simulink model "KPA_ALL"  (R2022b)
settings: Solver=FixedStepAuto  StartTime=0.0  StopTime=1  RelTol=1e-3
model workspace (MAT data in the model file):
  OutputBufferSize = 2
  OutputSampesPerSymbol = 4
  OutputSamplesPerSymbol = 4
  SNR = 16
  SampleTimeGenerator = 2.5e-06
undefined symbols (not defined in the file or in its folder): Add, DiscIntNeverNeededParam, magnitude, Shift
libraries: hdlsllib x16, simulink x5, commhdlcrc x3, commdigbbndpm3 x2, commfilt2 x2, commdigbbndam3 x2, commchan3 x1, commseqgen3 x1, commrandsrc3 x1, commsync2 x1, commsink2 x1, commutil2 x1
(part 1 of 2)
settings Model: Creator=Federal_PC  LastModifiedBy=svdvl
settings DebuggingCC: UnconnectedInputMsg=warning  UnconnectedOutputMsg=warning  UnconnectedLineMsg=warning
settings ModelReferenceCC: EnableRefExpFcnMdlSchedulingChecks=on
settings RTWCC: DLArmComputeVersion=19.05

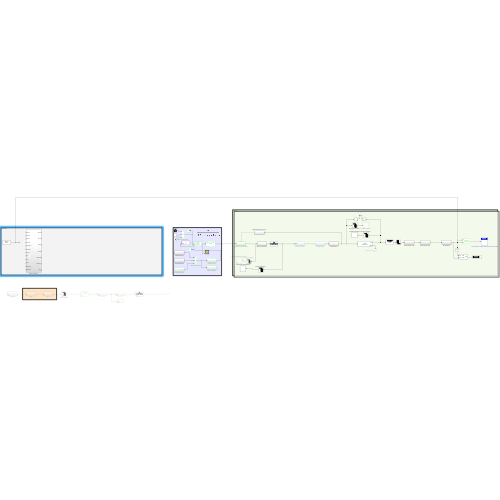
[thumbnail: Simulink's stored preview of the top-level diagram]
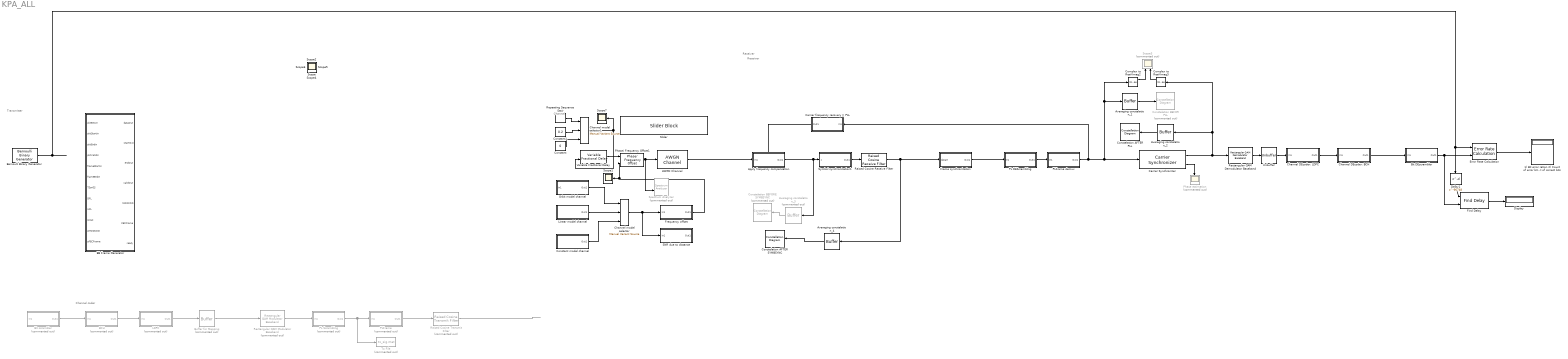
== system KPA_ALL ==
  note: Receiver
  note: Transmitter
  note: Channel
  note: Receiver
  note: Channel coder
  1) Bit error ration 2) Count of error bits 3) count of correct bits : Display
  AWGN Channel : commchan3/AWGN Channel  InputProcessing=Columns as channels (frame based)  seed=67  noiseMode="Signal to noise ratio  (SNR)"  EbNodB=15  EsNodB=10  SNRdB=SNR + 10*log10(4)  bitsPerSym=1  Ps=1  Tsym=1  variance=1
  Apply frequency compensation : Subsystem
  Averaging constelation_1 : Buffer  N=100  OutputFrames=off
  Averaging constelation_2 : Buffer  N=100  OutputFrames=off
  Averaging constelation_3 : Buffer  Commented=on  N=100  OutputFrames=off
  Averaging constelation_4 : Buffer  N=100  OutputFrames=off
  BB Frame Generator : Subsystem
  BCH : Subsystem  Commented=on
  Bernoulli Binary Generator : commrandsrc3/Bernoulli Binary Generator  ProbabilityOfZero=0.5  SeedSource=Auto  Seed=0  SampleTime=SampleTimeGenerator  SamplesPerFrame=1  OutputDataType=double  SimulateUsing=Interpreted execution
  Bit DEscrambler : Subsystem
  Bit scrambler : Subsystem  Commented=on
  Buffer for Mapping : Buffer  Commented=on  N=OutputBufferSize  OutputFrames=off
  Carrier Synchronizer : commsync2/Carrier Synchronizer  Modulation=QAM  ModulationPhaseOffset=Auto  CustomPhaseOffset=3*pi/2  SamplesPerSymbol=4  DampingFactor=0.707  NormalizedLoopBandwidth=0.01  EstimatedPhaseErrorOutputPort=on  SimulateUsing=Code generation
  Carrier frequency recovery || PLL : Subsystem
  Channel DEcoder: BCH : Subsystem
  Channel DEcoder: LDPC : Subsystem
  Channel model selector : simulink/Signal Routing/Manual Variant Source  NumChoices=3  LabelModeActiveChoice=V_3
  Channel model selector1 : simulink/Signal Routing/Manual Variant Source  NumChoices=3  LabelModeActiveChoice=V_2
  Complex to Real-Imag2 : ComplexToRealImag
  Complex to Real-Imag3 : ComplexToRealImag
  Constant : Constant  Value=0  SampleTime=-1
  Constant model channel : Subsystem
  Constant1 : Constant  Value=0.2  SampleTime=-1
  Constelation AFTER PLL : ConstellationDiagram  WindowPosition=[236.000000,590.000000,607.000000,426.000000,]  ScopeFrameLocation=window  XLimits=[-1.3206 1.3204]  YLimits=[-1.3206 1.3204]  DefaultConfigurationName=comm.scopes.ConstellationDiagramBlockCfg
  Constelation AFTER SYMBSYNC : ConstellationDiagram  WindowPosition=[598.000000,47.000000,607.000000,426.000000,]  ScopeFrameLocation=window  XLimits=[-1.3206 1.3204]  YLimits=[-1.3206 1.3204]  DefaultConfigurationName=comm.scopes.ConstellationDiagramBlockCfg
  Constelation BEFOR PLL : ConstellationDiagram  Commented=on  WindowPosition=[144 65 607 426]  XLimits=[-1.3197 1.321]  YLimits=[-1.3197 1.321]  ShowTrajectory=on  DefaultConfigurationName=comm.scopes.ConstellationDiagramBlockCfg
  Constelation BEFORE SYMBSYNC : ConstellationDiagram  Commented=on  WindowPosition=[233.000000,127.000000,607.000000,430.000000,]  ScopeFrameLocation=window  XLimits=[-1.3206 1.3204]  YLimits=[-1.3206 1.3204]  DefaultConfigurationName=comm.scopes.ConstellationDiagramBlockCfg
  Delay1 : Delay  DelayLength=96748
  Display : Display
  Error Rate Calculation : commsink2/Error Rate Calculation  N=96748+4  st_delay=0  cp_mode=Entire frame  subframe=[]  PMode=Port  WsName=ErrorVec  RsMode2=off  stop=off  numErr=100  maxBits=1e6
  Find Delay : commutil2/Find Delay  corrLength=100  chgSigOP=off  stopUpdate=off  numConstDelay=3
  Frame synchronization : Subsystem
  Frequency offset : Subsystem
  LDPC : Subsystem  Commented=on
  Linear model channel : Subsystem
  Orbit model channel : Subsystem
  PL DEScrambling : Subsystem
  PL Scrambling : Subsystem  Commented=on
  PLFrame : Subsystem  Commented=on
  PLFrame demux : Subsystem
  Phase estimation : Scope  Commented=on
  Phase/ Frequency Offset1 : commrflib2/Phase// Frequency Offset  phaseOffset=0  freqPort=on  freqOffset=3
  Raised Cosine Receive Filter : commfilt2/Raised Cosine Receive Filter  filtType=Square root  R=0.2  filtSpan=20  N=2  downFactor=2  downOffset=0  filterGain=1  RateOptions=Allow multirate processing  framing=Mute  checkCoeff=off  variableName=rcRxFilt  currentFiltSpan=10  D=5  inputOffset=0  sampMode=Mute  saveAsFlag=0  rateMode=Downsampling  checkGain=Normalized  launchFVT=on  roundingMode=Floor  overflowMode=off  coeffDataTypeStr=Inherit: Same word length as input  coeffMin=[]  coeffMax=[]  coeffLastDataTypeStr=Inherit: Same word length as input  accumDataTypeStr=Inherit: Same as product output  accumLastDataTypeStr=Inherit: Same as product output  outputDataTypeStr=Inherit: Same as accumulator  outputMin=[]  outputMax=[]  outputLastDataTypeStr=Inherit: Same as accumulator
  Raised Cosine Transmit Filter : commfilt2/Raised Cosine Transmit Filter  Commented=on  filtType=Square root  R=0.2  filtSpan=20  N=2  filterGain=1  RateOptions=Allow multirate processing  framing=Mute  checkCoeff=off  variableName=rcTxFilt  checkGain=Normalized  sampMode=Mute  saveAsFlag=0  currentFiltSpan=10  D=5  launchFVT=on  roundingMode=Floor  overflowMode=off  coeffDataTypeStr=Inherit: Same word length as input  coeffMin=[]  coeffMax=[]  coeffLastDataTypeStr=Inherit: Same word length as input  outputDataTypeStr=Inherit: Same as accumulator  outputMin=[]  outputMax=[]  outputLastDataTypeStr=Inherit: Same as accumulator
  Rectangular QAM Demodulator Baseband : commdigbbndam3/Rectangular QAM Demodulator Baseband  M=4  OutType=Bit  DecType=Hard decision  VarSource=Dialog  Variance=1  Dec=Gray  Mapping=[0:15]  PowType=Min. distance between symbols  MinDist=2  AvgPow=1  PeakPow=1  Ph=0  outDtype1=Inherit via internal rule  outDtype2=Inherit via internal rule  derotateFactorDTMode=Specify word length  derotateFactorWordLen=16  derotateFactorDataTypeStr=fixdt(1,16)  derotateFactorLastDataTypeStr=fixdt(1,16)  denormFactorWordLen=16  denormFactorDataTypeStr=Inherit: Same word length as input  denormFactorLastDataTypeStr=Inherit: Same word length as input  prodOutWordLen=32  prodOutOverflowMode=Wrap  prodOutRoundingMode=Floor  prodOutOvFlMode=off  prodOutOvFlModeLastStrValue=off  sumWordLen=32
  Rectangular QAM Modulator Baseband : commdigbbndam3/Rectangular QAM Modulator Baseband  Commented=on  M=4  InType=Bit  Enc=Gray  Mapping=[0:15]  PowType=Average Power  MinDist=2  AvgPow=1  PeakPow=1  Ph=0  outDtype=double  outWordLen=16  outUDDataType=sfix(16)  outFracLenMode=Best precision  outFracLen=15  outDataTypeStr=double  outLastDataTypeStr=double
  Repeating Sequence Stair : simulink/Sources/Repeating Sequence Stair  OutValues=[0:0.1:0.9 0.8:-0.1:0.1]  tsamp=-1  OutMin=[]  OutMax=[]  OutDataTypeStr=double  OutputDataTypeScalingMode=double  OutDataType=fixdt(0,8)  ConRadixGroup=Best Precision: Vector-wise  OutScaling=2^-12
  SNR due to distance : Subsystem
  Scope{,1..2,4..7} (7 alike) : Scope
  Scope3 : Scope  Commented=on  NumInputPorts=2
  Slider : SliderBlock  ScaleMin=-10  ScaleMax=50  TickInterval=5
  Spectrum Analyzer : SpectrumAnalyzer  Commented=on  NumInputPorts=2
  Symbol synchronization1 : Subsystem
  To File : ToFile  Commented=on  Filename=tx_sig.mat  SaveFormat=Timeseries
  Unbuffer : Unbuffer
  Variable Fractional Delay : dspsigops/Variable Fractional Delay  mode=OBSOLETE  modeActive=Linear  L=4  FarrowL=4  R=10  alpha=1  dmax=100  ic=0  noDFT=off  fallbackFIR=Clip to the minimum value necessary for centered kernel  fallbackFarrow=Clip to the minimum value necessary for centered kernel  roundingMode=Zero  overflowMode=off
  wires:
  Phase/ Frequency Offset1/1 -> Spectrum Analyzer/2, AWGN Channel/1
  Complex to Real-Imag2/1 -> Scope3/1
  Complex to Real-Imag3/1 -> Scope3/2
  Averaging constelation_2/1 -> Constelation AFTER PLL/1
  Carrier Synchronizer/1 -> Rectangular QAM Demodulator Baseband/1, Complex to Real-Imag3/1, Averaging constelation_2/1
  Carrier Synchronizer/2 -> Phase estimation/1
  Averaging constelation_1/1 -> Constelation BEFOR PLL/1
  Orbit model channel/1(Out1) -> Channel model selector/1
  Linear model channel/1(Out1) -> Channel model selector/2
  Constant model channel/1(Out1) -> Channel model selector/3
  Channel model selector/1 -> Frequency offset/1(In1), SNR due to distance/1(In1)
  Frequency offset/1(Out1) -> Phase/ Frequency Offset1/2, Scope1/1
  PLFrame demux/1(Out1) -> Carrier frequency recovery || PLL/1(In1), Complex to Real-Imag2/1, Averaging constelation_1/1, Carrier Synchronizer/1
  Carrier frequency recovery || PLL/1(Out1) -> ?
  PL DEScrambling/1(Out1) -> PLFrame demux/1(In1)
  Channel DEcoder: LDPC/1(Out1) -> Channel DEcoder: BCH/1(In1)
  Bit DEscrambler/1(Out1) -> Find Delay/2, Error Rate Calculation/2
  Rectangular QAM Demodulator Baseband/1 -> Unbuffer/1
  Bernoulli Binary Generator/1 -> Delay1/1, Error Rate Calculation/1
  Error Rate Calculation/1 -> 1) Bit error ration 2) Count of error bits 3) count of correct bits/1
  AWGN Channel/1 -> Apply frequency compensation/1(In1)
  Find Delay/1 -> Display/1
  Unbuffer/1 -> Channel DEcoder: LDPC/1(In1)
  Delay1/1 -> Find Delay/1
  Channel DEcoder: BCH/1(Out1) -> Bit DEscrambler/1(In1)
  Variable Fractional Delay/1 -> Phase/ Frequency Offset1/1
  Averaging constelation_3/1 -> Constelation BEFORE SYMBSYNC/1
  Repeating Sequence Stair/1 -> Channel model selector1/1
  Channel model selector1/1 -> Scope7/1, Variable Fractional Delay/2
  Constant/1 -> Channel model selector1/3
  Constant1/1 -> Channel model selector1/2
  Apply frequency compensation/1(Out1) -> Symbol synchronization1/1(x), Averaging constelation_3/1
  Averaging constelation_4/1 -> Constelation AFTER SYMBSYNC/1
  Frame synchronization/1(Out1) -> PL DEScrambling/1(In1)
  Symbol synchronization1/1(Out1) -> Raised Cosine Receive Filter/1
  Raised Cosine Receive Filter/1 -> Averaging constelation_4/1, Frame synchronization/1(dataIn)
  PLFrame/1(Out1) -> Raised Cosine Transmit Filter/1
  PL Scrambling/1(Out1) -> To File/1, PLFrame/1(In1)
  Raised Cosine Transmit Filter/1 -> ?
  Rectangular QAM Modulator Baseband/1 -> PL Scrambling/1(In1)
  LDPC/1(Out1) -> Buffer for Mapping/1
  BCH/1(Out1) -> LDPC/1(In1)
  Buffer for Mapping/1 -> Rectangular QAM Modulator Baseband/1
  Bit scrambler/1(Out1) -> BCH/1(In1)

== system KPA_ALL/Apply frequency compensation ==
  In1 : Inport
  Out1 : Outport
  wires:
  In1/1 -> Out1/1

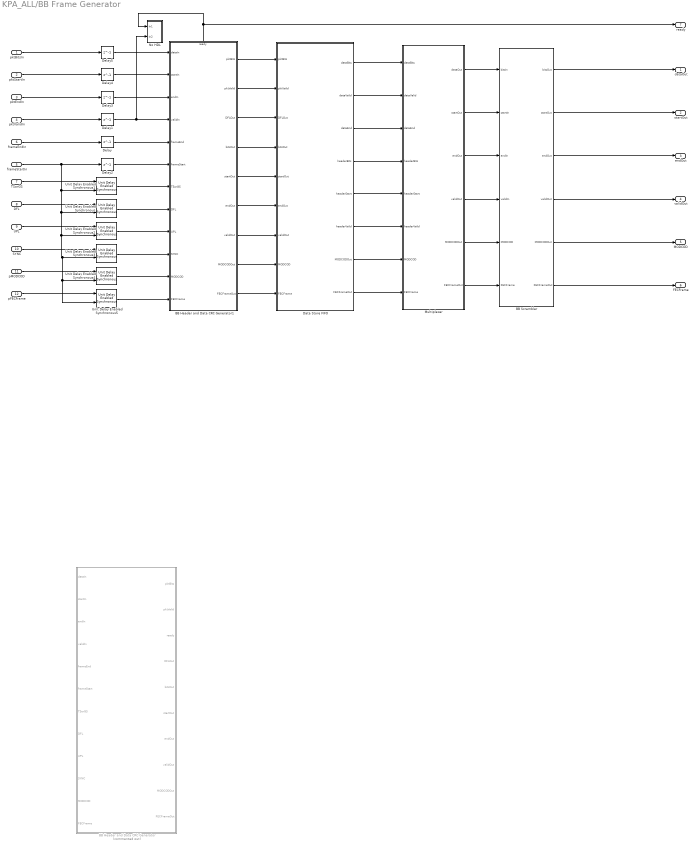
== system KPA_ALL/BB Frame Generator ==
  pktBitsIn : Inport
  pktStartIn : Inport  Port=2
  pktEndIn : Inport  Port=3
  pktValidIn : Inport  Port=4
  frameStartIn : Inport  Port=5
  frameEndIn : Inport  Port=6
  TSorGS : Inport  Port=7
  DFL : Inport  Port=8
  UPL : Inport  Port=9
  SYNC : Inport  Port=10
  pMODCOD : Inport  Port=11
  pFECFrame : Inport  Port=12
  BB Header and Data CRC Generator : Subsystem  Commented=on
  BB Header and Data CRC Generator1 : Subsystem
      settings: PortSchema="{\"entries\":[{\"content\":{\"sides\":[{\"content\":{\"connectorIds\":[\"In1\",\"In2\",\"In3\",\"In4\",\"In5\",\"In6\",\"In7\",\"In8\",\"In9\",\"In10\",\"In11\",\"In12\"]},\"type\":\"ConnectorPlacement.EquallySpacedRectSide\",\"uuid\":\"3add2032-9d60-4d0f-9380-dd456938382c\"},{\"content\":{\"connectorIds\":[\"Out1\",\"Out2\",\"Out3\",\"Out4\",\"Out5\",\"Out6\",\"Out7\",\"Out8\",\"Out9\"],\"side\":\"RIGHT\"},\"type\":\"ConnectorPlacement.EquallySpacedRectSide\",\"uuid\":\"1bf7c2ec-87b6-4e75-9963-e9b94fb225d2\"},{\"content\":{\"connectorIds\":[\"Out10\"],\"side\":\"TOP\"},\"type\":\"ConnectorPlacement.EquallySpacedRectSide\",\"uuid\":\"ca70afd1-66c9-458c-a276-a3db39240c3a\"}]},\"type\":\"ConnectorPlacement.EquallySpacedConnector\",\"uuid\":\"2d2892fe-640d-476a-8e13-3394180d2ea7\"}],\"packageUris\":[\"http://schema.mathworks.com/mf0/Connector/R2020b\"],\"version\":\"1.0\"}"
  BB Scrambler : Subsystem
  Data Store FIFO : Subsystem
  Delay{,1..5} (6 alike) : Delay  DelayLength=1
  Multiplexer : Subsystem
  No HDL : Subsystem
  Unit Delay Enabled Synchronous{,1..5} (6 alike) : hdlsllib/Discrete/Unit Delay Enabled Synchronous  InitialCondition=0.0  SampleTime=-1
  dataOut : Outport
  startOut : Outport  Port=2
  endOut : Outport  Port=3
  validOut : Outport  Port=4
  MODCOD : Outport  Port=5
  FECFrame : Outport  Port=6
  ready : Outport  Port=7
  wires:
  BB Header and Data CRC Generator1/6(endOut) -> Data Store FIFO/6(endOut)
  BB Header and Data CRC Generator1/7(validOut) -> Data Store FIFO/7(validOut)
  Delay/1 -> BB Header and Data CRC Generator1/5(frameEnd)
  BB Scrambler/3(endOut) -> endOut/1
  Multiplexer/4(validOut) -> BB Scrambler/4(validIn)
  Multiplexer/3(endOut) -> BB Scrambler/3(endIn)
  BB Header and Data CRC Generator1/2(pktValid) -> Data Store FIFO/2(pktValid)
  Data Store FIFO/6(headerValid) -> Multiplexer/6(headerValid)
  Data Store FIFO/2(dataValid) -> Multiplexer/2(dataValid)
  BB Header and Data CRC Generator1/4(bitsOut) -> Data Store FIFO/4(bitsOut)
  Data Store FIFO/3(dataEnd) -> Multiplexer/3(dataEnd)
  Delay2/1 -> BB Header and Data CRC Generator1/6(frameStart)
  BB Scrambler/2(startOut) -> startOut/1
  Delay4/1 -> BB Header and Data CRC Generator1/2(startIn)
  Unit Delay Enabled Synchronous/1 -> BB Header and Data CRC Generator1/8(DFL)
  DFL/1 -> Unit Delay Enabled Synchronous/1
  frameEndIn/1 -> Delay/1
  pktEndIn/1 -> Delay3/1
  TSorGS/1 -> Unit Delay Enabled Synchronous1/1
  pktBitsIn/1 -> Delay5/1
  BB Scrambler/6(FECFrameOut) -> FECFrame/1
  Delay1/1 -> No HDL/2(In2), BB Header and Data CRC Generator1/4(validIn)
  Multiplexer/6(FECFrameOut) -> BB Scrambler/6(FECFrame)
  Unit Delay Enabled Synchronous2/1 -> BB Header and Data CRC Generator1/9(UPL)
  BB Header and Data CRC Generator1/3(DFLOut) -> Data Store FIFO/3(DFLOut)
  Delay5/1 -> BB Header and Data CRC Generator1/1(dataIn)
  Data Store FIFO/1(dataBits) -> Multiplexer/1(dataBits)
  frameStartIn/1 -> Unit Delay Enabled Synchronous5/2, Unit Delay Enabled Synchronous4/2, Unit Delay Enabled Synchronous3/2, Unit Delay Enabled Synchronous2/2, Unit Delay Enabled Synchronous/2, Unit Delay Enabled Synchronous1/2, Delay2/1
  Data Store FIFO/8(FECFrameOut) -> Multiplexer/8(FECFrame)
  BB Header and Data CRC Generator1/9(FECFrameOut) -> Data Store FIFO/9(FECFrame)
  Multiplexer/1(dataOut) -> BB Scrambler/1(bitsIn)
  Unit Delay Enabled Synchronous3/1 -> BB Header and Data CRC Generator1/10(SYNC)
  Unit Delay Enabled Synchronous5/1 -> BB Header and Data CRC Generator1/12(FECFrame)
  Data Store FIFO/7(MODCODOut) -> Multiplexer/7(MODCOD)
  BB Scrambler/1(bitsOut) -> dataOut/1
  Multiplexer/2(startOut) -> BB Scrambler/2(startIn)
  pMODCOD/1 -> Unit Delay Enabled Synchronous4/1
  Delay3/1 -> BB Header and Data CRC Generator1/3(endIn)
  pktValidIn/1 -> Delay1/1
  Data Store FIFO/4(headerBits) -> Multiplexer/4(headerBits)
  BB Header and Data CRC Generator1/10(ready) -> ready/1, No HDL/1(In1)
  SYNC/1 -> Unit Delay Enabled Synchronous3/1
  BB Header and Data CRC Generator1/5(startOut) -> Data Store FIFO/5(startOut)
  BB Scrambler/5(MODCODOut) -> MODCOD/1
  pFECFrame/1 -> Unit Delay Enabled Synchronous5/1
  BB Scrambler/4(validOut) -> validOut/1
  UPL/1 -> Unit Delay Enabled Synchronous2/1
  pktStartIn/1 -> Delay4/1
  Data Store FIFO/5(headerStart) -> Multiplexer/5(headerStart)
  Unit Delay Enabled Synchronous4/1 -> BB Header and Data CRC Generator1/11(MODCOD)
  Unit Delay Enabled Synchronous1/1 -> BB Header and Data CRC Generator1/7(TSorGS)
  BB Header and Data CRC Generator1/1(pktBits) -> Data Store FIFO/1(pktBits)
  Multiplexer/5(MODCODOut) -> BB Scrambler/5(MODCOD)
  BB Header and Data CRC Generator1/8(MODCODOut) -> Data Store FIFO/8(MODCOD)

== system KPA_ALL/BCH ==
  In1 : Inport
  Out1 : Outport
  wires:
  In1/1 -> Out1/1

== system KPA_ALL/Bit DEscrambler ==
  In1 : Inport
  Out1 : Outport
  wires:
  In1/1 -> Out1/1

== system KPA_ALL/Bit scrambler ==
  In1 : Inport
  Out1 : Outport
  wires:
  In1/1 -> Out1/1

== system KPA_ALL/Carrier frequency recovery || PLL ==
  In1 : Inport
  Out1 : Outport
  wires:
  In1/1 -> Out1/1

== system KPA_ALL/Channel DEcoder: BCH ==
  In1 : Inport
  Out1 : Outport
  wires:
  In1/1 -> Out1/1

== system KPA_ALL/Channel DEcoder: LDPC ==
  In1 : Inport
  Out1 : Outport
  wires:
  In1/1 -> Out1/1

== system KPA_ALL/Constant model channel ==
  Constant : Constant  Value=0  SampleTime=-1
  Out1 : Outport
  wires:
  Constant/1 -> Out1/1

== system KPA_ALL/Frame synchronization ==
  dataIn : Inport
  Correlator : Subsystem
  Terminator : Terminator
  Out1 : Outport
  wires:
  dataIn/1 -> Out1/1, Correlator/1(dataIn)
  Correlator/1(SOFCorrOut) -> Terminator/1

== system KPA_ALL/Frequency offset ==
  In1 : Inport
  Out1 : Outport
  wires:
  In1/1 -> Out1/1

== system KPA_ALL/LDPC ==
  In1 : Inport
  Out1 : Outport
  wires:
  In1/1 -> Out1/1

== system KPA_ALL/Linear model channel ==
  Constant : Constant  SampleTime=SampleTimeGenerator*OutputBufferSize/OutputSamplesPerSymbol
  Discrete-Time Integrator : DiscreteIntegrator  gainval=10000  SampleTime=-1  ICPrevOutput=DiscIntNeverNeededParam  ICPrevScaledInput=DiscIntNeverNeededParam
  Freq offset : Display
  Out1 : Outport
  wires:
  Constant/1 -> Discrete-Time Integrator/1
  Discrete-Time Integrator/1 -> Out1/1, Freq offset/1

== system KPA_ALL/Orbit model channel ==
  In1 : Inport
  Out1 : Outport
  wires:
  In1/1 -> Out1/1

== system KPA_ALL/PL DEScrambling ==
  In1 : Inport
  Out1 : Outport
  wires:
  In1/1 -> Out1/1

== system KPA_ALL/PL Scrambling ==
  In1 : Inport
  Out1 : Outport
  wires:
  In1/1 -> Out1/1

== system KPA_ALL/PLFrame ==
  In1 : Inport
  BPSK Modulator Baseband : commdigbbndpm3/BPSK Modulator Baseband  Ph=0  outDtype=double  outWordLen=16  outUDDataType=sfix(16)  outFracLenMode=Best precision  outFracLen=15  outDataTypeStr=double  outLastDataTypeStr=double
  Buffer : Buffer  N=16110  OutputFrames=off
  Constant : Constant  Value=[0 1 1 0 0 0 1 1 0 1 0 0 1 0 1 1 1 0 1 0 0 0 0 0 1 0 0 1 1 1 0 0 0 1 1 0 0 1 1 1 0 1 1 0 0 0 0 0 1 1 1 1 0 0 1 0 0 1 0 1 0 1 0 0 1 1 0 1 0 0 0 0 1 0 0 0 1 0 1 1 0 1 1 1 1 1 1 0 1 0]  SampleTime=-1
  Gain : Gain
  Unbuffer : Unbuffer  ic=16200
  Vector Concatenate : Concatenate
  Out1 : Outport
  wires:
  Vector Concatenate/1 -> Unbuffer/1
  Buffer/1 -> Vector Concatenate/2
  In1/1 -> Buffer/1
  Unbuffer/1 -> Out1/1
  Gain/1 -> Vector Concatenate/1
  BPSK Modulator Baseband/1 -> Gain/1
  Constant/1 -> BPSK Modulator Baseband/1

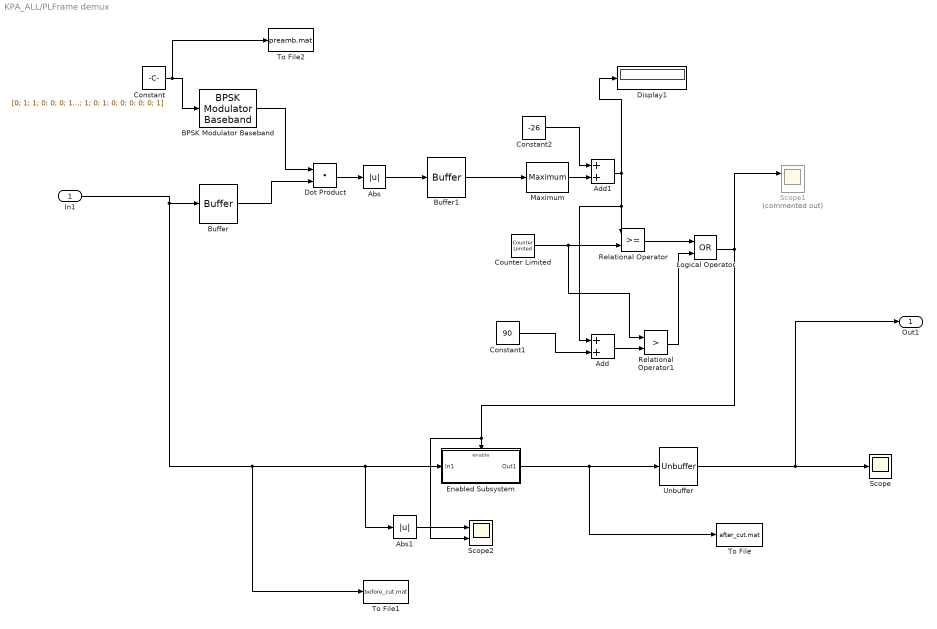
== system KPA_ALL/PLFrame demux ==
  In1 : Inport
  Abs : Abs  SaturateOnIntegerOverflow=off
  Abs1 : Abs  SaturateOnIntegerOverflow=off
  Add : Sum
  Add1 : Sum
  BPSK Modulator Baseband : commdigbbndpm3/BPSK Modulator Baseband  Ph=0  outDtype=double  outWordLen=16  outUDDataType=sfix(16)  outFracLenMode=Best precision  outFracLen=15  outDataTypeStr=double  outLastDataTypeStr=double
  Buffer : Buffer  N=25  V=24  OutputFrames=off
  Buffer1 : Buffer  N=16200  OutputFrames=off
  Constant : Constant  Value=[0; 1; 1; 0; 0; 0; 1; 1; 0; 1; 0; 0; 1; 0; 1; 1; 1; 0; 1; 0; 0; 0; 0; 0; 1]  SampleTime=-1
  Constant1 : Constant  Value=90  SampleTime=5e-6*16110/16200
  Constant2 : Constant  Value=-26  SampleTime=-1
  Counter Limited : hdlsllib/Sources/Counter Limited  uplimit=16200-1  tsamp=5e-6*16110/16200
  Display1 : Display
  Dot Product : DotProduct  OutDataTypeStr=Inherit: Inherit via internal rule
  Enabled Subsystem : Subsystem  TreatAsAtomicUnit=on
  Logical Operator : Logic  Operator=OR  AllPortsSameDT=off  OutDataTypeStr=boolean
  Maximum : dspstat3/Maximum  operation=maximum  fcn=Index  indexBase=One  operateOver=Each column  Dimension=1  InputProcessing=Columns as channels (frame based)  reset=None  roiEnable=off  roiType=Rectangles  roiPortion=Entire ROI  roiOutput=Individual statistics for each ROI  roiFlag=off  roundingMode=Floor  overflowMode=off  accumDataTypeStr=Inherit: Same as product output  accumLastDataTypeStr=Inherit: Same as product output
  Relational Operator : RelationalOperator  OutDataTypeStr=boolean  InputSameDT=off
  Relational Operator1 : RelationalOperator  Operator=>  OutDataTypeStr=boolean  InputSameDT=off
  Scope : Scope
  Scope1 : Scope  Commented=on  NumInputPorts=2
  Scope2 : Scope  NumInputPorts=2
  To File : ToFile  Filename=after_cut.mat  SaveFormat=Timeseries
  To File1 : ToFile  Filename=before_cut.mat  SaveFormat=Timeseries
  To File2 : ToFile  Filename=preamb.mat  SaveFormat=Timeseries
  Unbuffer : Unbuffer
  Out1 : Outport
  wires:
  Constant/1 -> To File2/1, BPSK Modulator Baseband/1
  Buffer/1 -> Dot Product/2
  Dot Product/1 -> Abs/1
  BPSK Modulator Baseband/1 -> Dot Product/1
  Abs/1 -> Buffer1/1
  Buffer1/1 -> Maximum/1
  Counter Limited/1 -> Relational Operator1/1, Relational Operator/2
  Relational Operator/1 -> Logical Operator/1
  Constant1/1 -> Add/2
  Add/1 -> Relational Operator1/2
  Relational Operator1/1 -> Logical Operator/2
  Enabled Subsystem/1(Out1) -> To File/1, Unbuffer/1
  Unbuffer/1 -> Scope/1, Out1/1
  Abs1/1 -> Scope2/1
  Logical Operator/1 -> Scope2/2, Enabled Subsystem/Enable, Scope1/1
  In1/1 -> Abs1/1, Enabled Subsystem/1(In1), To File1/1, Buffer/1
  Maximum/1 -> Add1/2
  Constant2/1 -> Add1/1
  Add1/1 -> Display1/1, Add/1, Relational Operator/1

== system KPA_ALL/SNR due to distance ==
  In1 : Inport
  Out1 : Outport
  wires:
  In1/1 -> Out1/1

== system KPA_ALL/Symbol synchronization1 ==
  x : Inport
  Constant : Constant  Value=-0.1
  Constant1 : Constant  Value=-1
  Interpolation control : Subsystem
  Linear Interpolator : Subsystem
      settings: PortSchema="{\"entries\":[{\"content\":{\"sides\":[{\"content\":{\"connectorIds\":[\"In1\"]},\"type\":\"ConnectorPlacement.EquallySpacedRectSide\",\"uuid\":\"e185856d-5f81-4c71-aeba-8657e8be69b7\"},{\"content\":{\"connectorIds\":[\"Out1\"],\"side\":\"RIGHT\"},\"type\":\"ConnectorPlacement.EquallySpacedRectSide\",\"uuid\":\"487ec109-4505-4025-a071-939a946bead6\"},{\"content\":{\"connectorIds\":[\"In2\"],\"side\":\"TOP\"},\"type\":\"ConnectorPlacement.EquallySpacedRectSide\",\"uuid\":\"bdbbf84f-c060-4097-b440-093ef9dcf44f\"},{\"content\":{\"connectorIds\":[],\"side\":\"BOTTOM\"},\"type\":\"ConnectorPlacement.EquallySpacedRectSide\",\"uuid\":\"14959837-ab14-4ae0-ae0e-9624de46668b\"}]},\"type\":\"ConnectorPlacement.EquallySpacedConnector\",\"uuid\":\"80c256de-e921-4425-90d6-76c464211f17\"}],\"packageUris\":[\"http://schema.mathworks.com/mf0/Connector/R2020b\"],\"version\":\"1.0\"}"
  Loop filter : Subsystem
  Product : Product
  Scope : Scope
  TED : Subsystem
  TED selector : simulink/Signal Routing/Manual Variant Source  NumChoices=3  LabelModeActiveChoice=V_1
  Out1 : Outport
  wires:
  Loop filter/1(Out1) -> Interpolation control/1(In1)
  Linear Interpolator/1(Out1) -> Out1/1, TED/1(In1)
  x/1 -> Linear Interpolator/1(x)
  TED/1(Out1) -> Scope/1, Loop filter/1(In1)
  Constant/1 -> TED selector/2
  TED selector/1 -> Linear Interpolator/2(mu)
  Product/1 -> TED selector/1
  Interpolation control/1(mu) -> Product/1
  Constant1/1 -> Product/2

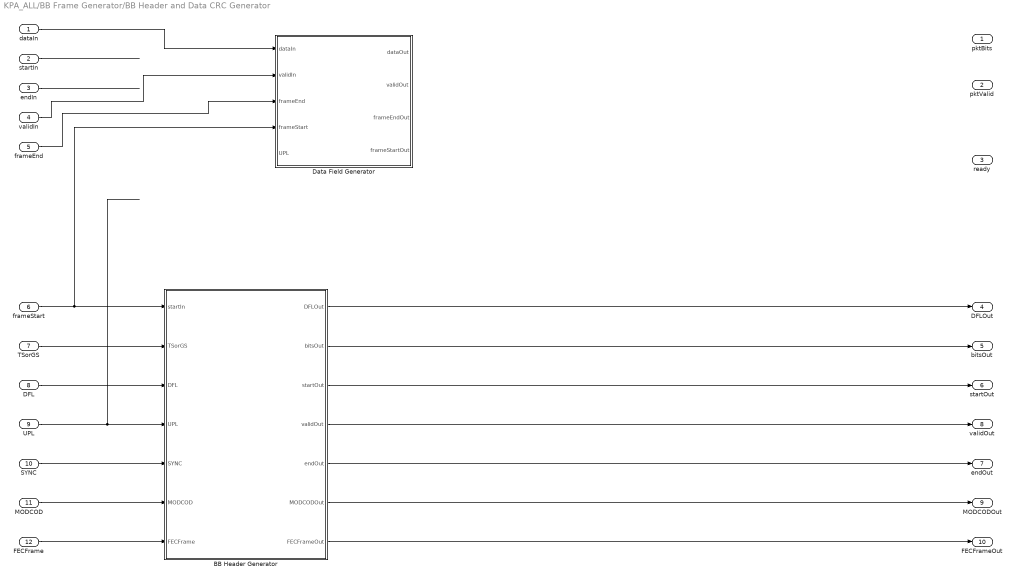
== system KPA_ALL/BB Frame Generator/BB Header and Data CRC Generator ==
  dataIn : Inport
  startIn : Inport  Port=2
  endIn : Inport  Port=3
  validIn : Inport  Port=4
  frameEnd : Inport  Port=5
  frameStart : Inport  Port=6
  TSorGS : Inport  Port=7
  DFL : Inport  Port=8
  UPL : Inport  Port=9
  SYNC : Inport  Port=10
  MODCOD : Inport  Port=11
  FECFrame : Inport  Port=12
  BB Header Generator : Subsystem
  Data Field Generator : Subsystem
  pktBits : Outport
  pktValid : Outport  Port=2
  ready : Outport  Port=3
  DFLOut : Outport  Port=4
  bitsOut : Outport  Port=5
  startOut : Outport  Port=6
  endOut : Outport  Port=7
  validOut : Outport  Port=8
  MODCODOut : Outport  Port=9
  FECFrameOut : Outport  Port=10
  wires:
  endIn/1 -> ?
  frameEnd/1 -> Data Field Generator/3(frameEnd)
  dataIn/1 -> Data Field Generator/1(dataIn)
  validIn/1 -> Data Field Generator/2(validIn)
  startIn/1 -> ?
  MODCOD/1 -> BB Header Generator/6(MODCOD)
  UPL/1 -> BB Header Generator/4(UPL)
  TSorGS/1 -> BB Header Generator/2(TSorGS)
  DFL/1 -> BB Header Generator/3(DFL)
  SYNC/1 -> BB Header Generator/5(SYNC)
  FECFrame/1 -> BB Header Generator/7(FECFrame)
  frameStart/1 -> Data Field Generator/4(frameStart), BB Header Generator/1(startIn)
  ? -> ready/1
  ? -> pktValid/1
  ? -> pktBits/1
  BB Header Generator/2(bitsOut) -> bitsOut/1
  BB Header Generator/6(MODCODOut) -> MODCODOut/1
  BB Header Generator/7(FECFrameOut) -> FECFrameOut/1
  BB Header Generator/5(endOut) -> endOut/1
  BB Header Generator/1(DFLOut) -> DFLOut/1
  BB Header Generator/3(startOut) -> startOut/1
  BB Header Generator/4(validOut) -> validOut/1

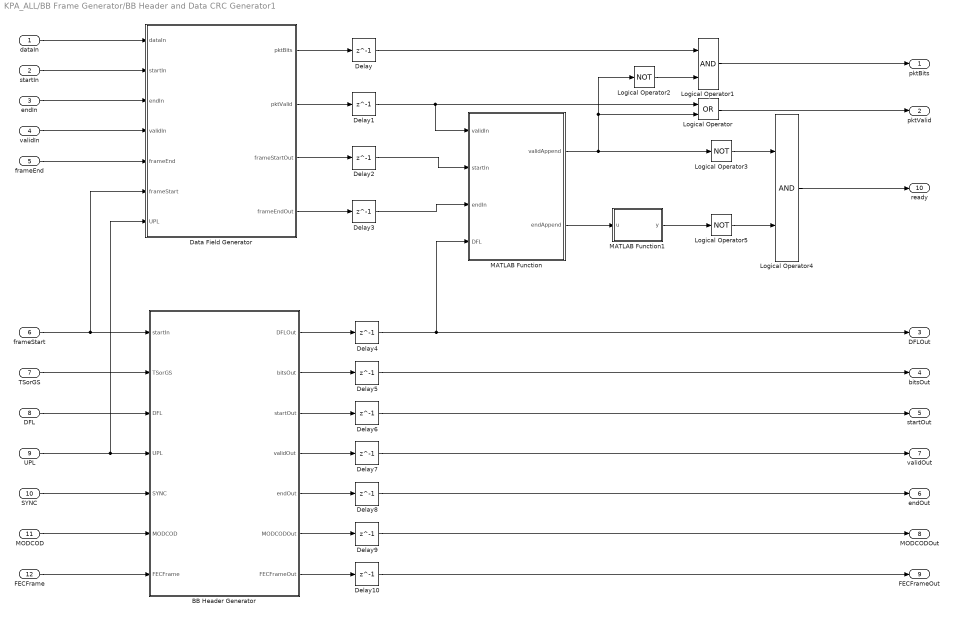
== system KPA_ALL/BB Frame Generator/BB Header and Data CRC Generator1 ==
  dataIn : Inport
  startIn : Inport  Port=2
  endIn : Inport  Port=3
  validIn : Inport  Port=4
  frameEnd : Inport  Port=5
  frameStart : Inport  Port=6
  TSorGS : Inport  Port=7
  DFL : Inport  Port=8
  UPL : Inport  Port=9
  SYNC : Inport  Port=10
  MODCOD : Inport  Port=11
  FECFrame : Inport  Port=12
  BB Header Generator : Subsystem
  Data Field Generator : Subsystem
  Delay{,1..10} (11 alike) : Delay  DelayLength=1
  Logical Operator : Logic  Operator=OR  AllPortsSameDT=off  OutDataTypeStr=boolean
  Logical Operator1 : Logic  AllPortsSameDT=off  OutDataTypeStr=boolean
  Logical Operator2 : Logic  Operator=NOT  AllPortsSameDT=off  OutDataTypeStr=boolean
  Logical Operator3 : Logic  Operator=NOT  AllPortsSameDT=off  OutDataTypeStr=boolean
  Logical Operator4 : Logic  AllPortsSameDT=off  OutDataTypeStr=boolean
  Logical Operator5 : Logic  Operator=NOT  AllPortsSameDT=off  OutDataTypeStr=boolean
  MATLAB Function : MATLAB Function  TreatAsAtomicUnit=on
  MATLAB Function1 : MATLAB Function  TreatAsAtomicUnit=on
  pktBits : Outport
  pktValid : Outport  Port=2
  DFLOut : Outport  Port=3
  bitsOut : Outport  Port=4
  startOut : Outport  Port=5
  endOut : Outport  Port=6
  validOut : Outport  Port=7
  MODCODOut : Outport  Port=8
  FECFrameOut : Outport  Port=9
  ready : Outport  Port=10
  wires:
  TSorGS/1 -> BB Header Generator/2(TSorGS)
  BB Header Generator/2(bitsOut) -> Delay5/1
  DFL/1 -> BB Header Generator/3(DFL)
  validIn/1 -> Data Field Generator/4(validIn)
  BB Header Generator/4(validOut) -> Delay7/1
  UPL/1 -> Data Field Generator/7(UPL), BB Header Generator/4(UPL)
  endIn/1 -> Data Field Generator/3(endIn)
  Data Field Generator/4(frameEndOut) -> Delay3/1
  startIn/1 -> Data Field Generator/2(startIn)
  dataIn/1 -> Data Field Generator/1(dataIn)
  BB Header Generator/3(startOut) -> Delay6/1
  frameStart/1 -> Data Field Generator/6(frameStart), BB Header Generator/1(startIn)
  SYNC/1 -> BB Header Generator/5(SYNC)
  frameEnd/1 -> Data Field Generator/5(frameEnd)
  BB Header Generator/5(endOut) -> Delay8/1
  BB Header Generator/1(DFLOut) -> Delay4/1
  Data Field Generator/2(pktValid) -> Delay1/1
  Data Field Generator/1(pktBits) -> Delay/1
  Data Field Generator/3(frameStartOut) -> Delay2/1
  MATLAB Function/1(validAppend) -> Logical Operator3/1, Logical Operator/2, Logical Operator2/1
  MATLAB Function/2(endAppend) -> MATLAB Function1/1(u)
  Logical Operator2/1 -> Logical Operator1/2
  Logical Operator1/1 -> pktBits/1
  Logical Operator3/1 -> Logical Operator4/1
  MATLAB Function1/1(y) -> Logical Operator5/1
  Logical Operator4/1 -> ready/1
  Logical Operator5/1 -> Logical Operator4/2
  Logical Operator/1 -> pktValid/1
  BB Header Generator/6(MODCODOut) -> Delay9/1
  MODCOD/1 -> BB Header Generator/6(MODCOD)
  Delay/1 -> Logical Operator1/1
  Delay1/1 -> MATLAB Function/1(validIn), Logical Operator/1
  Delay2/1 -> MATLAB Function/2(startIn)
  Delay3/1 -> MATLAB Function/3(endIn)
  Delay4/1 -> DFLOut/1, MATLAB Function/4(DFL)
  Delay5/1 -> bitsOut/1
  Delay6/1 -> startOut/1
  Delay7/1 -> validOut/1
  Delay8/1 -> endOut/1
  Delay9/1 -> MODCODOut/1
  FECFrame/1 -> BB Header Generator/7(FECFrame)
  BB Header Generator/7(FECFrameOut) -> Delay10/1
  Delay10/1 -> FECFrameOut/1

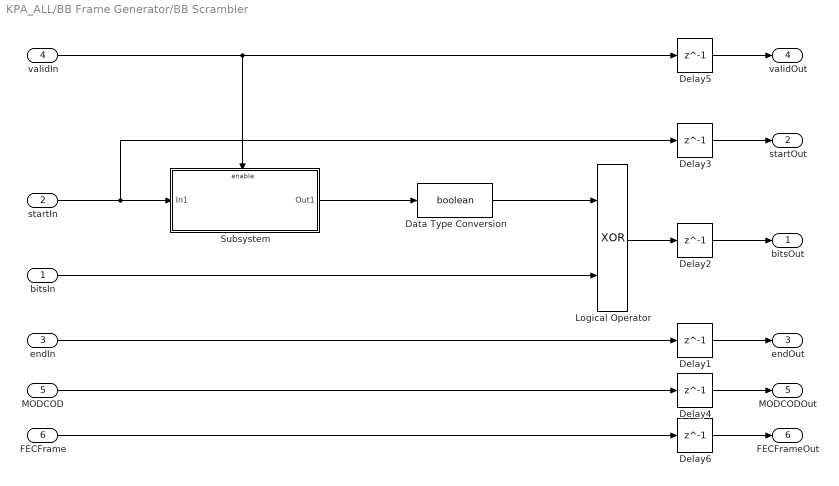
== system KPA_ALL/BB Frame Generator/BB Scrambler ==
  bitsIn : Inport
  startIn : Inport  Port=2
  endIn : Inport  Port=3
  validIn : Inport  Port=4
  MODCOD : Inport  Port=5
  FECFrame : Inport  Port=6
  Data Type Conversion : DataTypeConversion  OutDataTypeStr=boolean  SaturateOnIntegerOverflow=off  RndMeth=Floor
  Delay{1..6} (6 alike) : Delay  DelayLength=1
  Logical Operator : Logic  Operator=XOR  AllPortsSameDT=off  OutDataTypeStr=boolean
  Subsystem : Subsystem
  bitsOut : Outport
  startOut : Outport  Port=2
  endOut : Outport  Port=3
  validOut : Outport  Port=4
  MODCODOut : Outport  Port=5
  FECFrameOut : Outport  Port=6
  wires:
  endIn/1 -> Delay1/1
  bitsIn/1 -> Logical Operator/2
  validIn/1 -> Delay5/1, Subsystem/Enable
  Subsystem/1(Out1) -> Data Type Conversion/1
  startIn/1 -> Delay3/1, Subsystem/1(In1)
  Logical Operator/1 -> Delay2/1
  Data Type Conversion/1 -> Logical Operator/1
  MODCOD/1 -> Delay4/1
  Delay5/1 -> validOut/1
  Delay3/1 -> startOut/1
  Delay2/1 -> bitsOut/1
  Delay1/1 -> endOut/1
  Delay4/1 -> MODCODOut/1
  Delay6/1 -> FECFrameOut/1
  FECFrame/1 -> Delay6/1

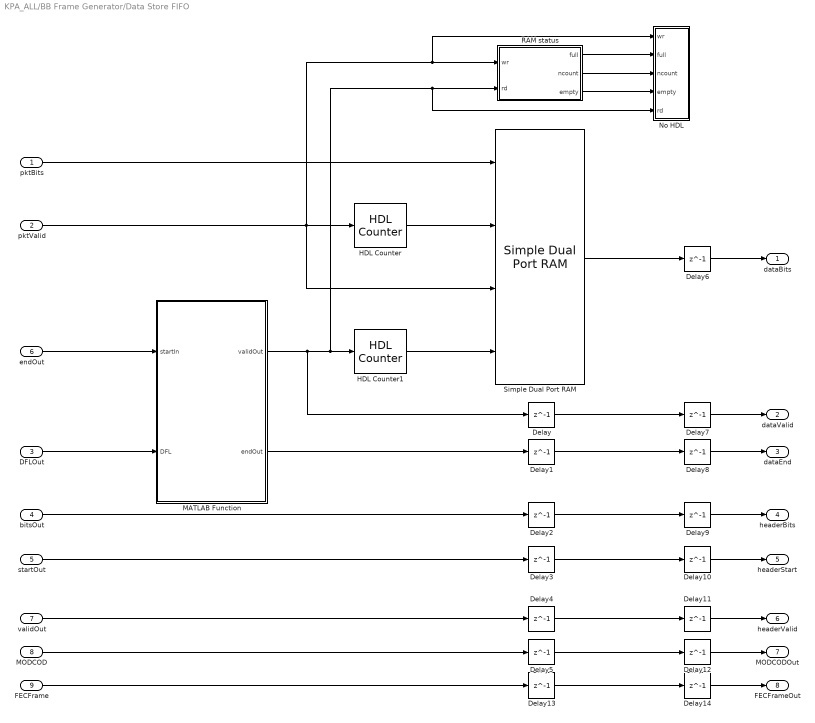
== system KPA_ALL/BB Frame Generator/Data Store FIFO ==
  pktBits : Inport
  pktValid : Inport  Port=2
  DFLOut : Inport  Port=3
  bitsOut : Inport  Port=4
  startOut : Inport  Port=5
  endOut : Inport  Port=6
  validOut : Inport  Port=7
  MODCOD : Inport  Port=8
  FECFrame : Inport  Port=9
  Delay{,1..14} (15 alike) : Delay  DelayLength=1
  HDL Counter : hdlsllib/Sources/HDL Counter  CountType=Count limited  CountInit=0  CountStep=1  CountMax=2^7-1  CountFromType=Initial value  CountFrom=0  CountResetPort=off  CountLoadPort=off  CountEnbPort=on  CountDirPort=off  CountHitOutputPort=off  CountDataType=Unsigned  CountWordLen=7  CountFracLen=0  CountSampTime=1
  HDL Counter1 : hdlsllib/Sources/HDL Counter  CountType=Count limited  CountInit=0  CountStep=1  CountMax=2^7-1  CountFromType=Initial value  CountFrom=0  CountResetPort=off  CountLoadPort=off  CountEnbPort=on  CountDirPort=off  CountHitOutputPort=off  CountDataType=Unsigned  CountWordLen=7  CountFracLen=0  CountSampTime=1
  MATLAB Function : MATLAB Function  TreatAsAtomicUnit=on
  No HDL : Subsystem
  RAM status : MATLAB Function  TreatAsAtomicUnit=on
  Simple Dual Port RAM : hdlsllib/HDL RAMs/Simple Dual Port RAM  ram_size=7
  dataBits : Outport
  dataValid : Outport  Port=2
  dataEnd : Outport  Port=3
  headerBits : Outport  Port=4
  headerStart : Outport  Port=5
  headerValid : Outport  Port=6
  MODCODOut : Outport  Port=7
  FECFrameOut : Outport  Port=8
  wires:
  endOut/1 -> MATLAB Function/1(startIn)
  pktBits/1 -> Simple Dual Port RAM/1
  pktValid/1 -> No HDL/1(wr), RAM status/1(wr), Simple Dual Port RAM/3, HDL Counter/1
  Simple Dual Port RAM/1 -> Delay6/1
  bitsOut/1 -> Delay2/1
  startOut/1 -> Delay3/1
  validOut/1 -> Delay4/1
  DFLOut/1 -> MATLAB Function/2(DFL)
  MATLAB Function/1(validOut) -> No HDL/5(rd), RAM status/2(rd), HDL Counter1/1, Delay/1
  HDL Counter1/1 -> Simple Dual Port RAM/4
  MATLAB Function/2(endOut) -> Delay1/1
  Delay/1 -> Delay7/1
  Delay1/1 -> Delay8/1
  Delay2/1 -> Delay9/1
  Delay4/1 -> Delay11/1
  HDL Counter/1 -> Simple Dual Port RAM/2
  Delay3/1 -> Delay10/1
  MODCOD/1 -> Delay5/1
  Delay5/1 -> Delay12/1
  Delay6/1 -> dataBits/1
  Delay7/1 -> dataValid/1
  Delay8/1 -> dataEnd/1
  Delay9/1 -> headerBits/1
  Delay10/1 -> headerStart/1
  Delay11/1 -> headerValid/1
  Delay12/1 -> MODCODOut/1
  FECFrame/1 -> Delay13/1
  Delay14/1 -> FECFrameOut/1
  Delay13/1 -> Delay14/1
  RAM status/3(empty) -> No HDL/4(empty)
  RAM status/2(ncount) -> No HDL/3(ncount)
  RAM status/1(full) -> No HDL/2(full)

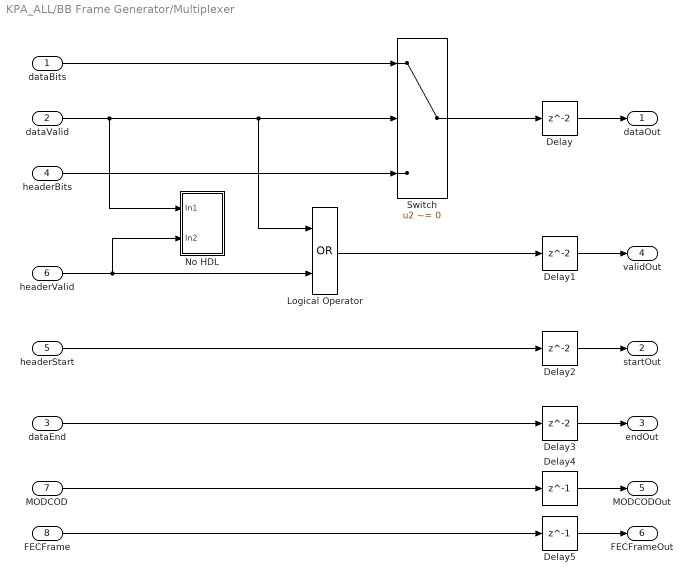
== system KPA_ALL/BB Frame Generator/Multiplexer ==
  dataBits : Inport
  dataValid : Inport  Port=2
  dataEnd : Inport  Port=3
  headerBits : Inport  Port=4
  headerStart : Inport  Port=5
  headerValid : Inport  Port=6
  MODCOD : Inport  Port=7
  FECFrame : Inport  Port=8
  Delay{,1..3} (4 alike) : Delay
  Delay4 : Delay  DelayLength=1
  Delay5 : Delay  DelayLength=1
  Logical Operator : Logic  Operator=OR  AllPortsSameDT=off  OutDataTypeStr=boolean
  No HDL : Subsystem
  Switch : Switch  Criteria=u2 ~= 0  SaturateOnIntegerOverflow=off  InputSameDT=off
  dataOut : Outport
  startOut : Outport  Port=2
  endOut : Outport  Port=3
  validOut : Outport  Port=4
  MODCODOut : Outport  Port=5
  FECFrameOut : Outport  Port=6
  wires:
  headerStart/1 -> Delay2/1
  dataEnd/1 -> Delay3/1
  dataBits/1 -> Switch/1
  headerBits/1 -> Switch/3
  headerValid/1 -> Logical Operator/2, No HDL/2(In2)
  Switch/1 -> Delay/1
  Logical Operator/1 -> Delay1/1
  MODCOD/1 -> Delay4/1
  dataValid/1 -> Switch/2, Logical Operator/1, No HDL/1(In1)
  Delay/1 -> dataOut/1
  Delay1/1 -> validOut/1
  Delay2/1 -> startOut/1
  Delay3/1 -> endOut/1
  Delay4/1 -> MODCODOut/1
  Delay5/1 -> FECFrameOut/1
  FECFrame/1 -> Delay5/1

== system KPA_ALL/BB Frame Generator/No HDL ==
  In1 : Inport
  In2 : Inport  Port=2
  Assertion : Assertion  StopWhenAssertionFail=off
  Logical Operator : Logic  AllPortsSameDT=off  OutDataTypeStr=boolean
  Logical Operator1 : Logic  Operator=NOT  AllPortsSameDT=off  OutDataTypeStr=boolean
  Logical Operator2 : Logic  Operator=NOT  AllPortsSameDT=off  OutDataTypeStr=boolean
  wires:
  Logical Operator1/1 -> Logical Operator/1
  In2/1 -> Logical Operator/2
  Logical Operator/1 -> Logical Operator2/1
  In1/1 -> Logical Operator1/1
  Logical Operator2/1 -> Assertion/1

== system KPA_ALL/Frame synchronization/Correlator ==
  note: Differential Detection
  dataIn : Inport
  Delay : Delay  DelayLength=1
  Math Function : Math  Operator=conj
  Product : Product  OutDataTypeStr=Inherit: Same as first input
  Scope : Scope
  SOFCorrOut : Outport
  wires:
  Math Function/1 -> Product/1
  Delay/1 -> Product/2
  dataIn/1 -> Delay/1, Math Function/1
  Product/1 -> Scope/1, SOFCorrOut/1

== system KPA_ALL/PLFrame demux/Enabled Subsystem ==
  In1 : Inport
  Enable : EnablePort
  Buffer : Buffer  N=16110  OutputFrames=off
  Rate Transition : RateTransition  Deterministic=off  OutPortSampleTime=0.08055
  Out1 : Outport  InitialOutput=0  VectorParamsAs1DForOutWhenUnconnected=off
  wires:
  In1/1 -> Buffer/1
  Buffer/1 -> Rate Transition/1
  Rate Transition/1 -> Out1/1

== system KPA_ALL/Symbol synchronization1/Interpolation control ==
  In1 : Inport
  mu : Outport
  wires:
  In1/1 -> mu/1

== system KPA_ALL/Symbol synchronization1/Linear Interpolator ==
  x : Inport
  mu : Inport  Port=2
  Buffer : Buffer  N=2  OutputFrames=off
  Constant : Constant  SampleTime=-1
  Product : Product
  Sum : Sum  Inputs=|+-
  Sum1 : Sum  Inputs=|-+
  Sum2 : Sum  Inputs=|++
  Unbuffer : Unbuffer
  Unit Delay : UnitDelay  SampleTime=-1  HasFrameUpgradeWarning=on
  Out1 : Outport
  wires:
  Unit Delay/1 -> Sum/2, Sum2/1
  Sum1/1 -> Product/2
  Sum/1 -> Product/1
  mu/1 -> Sum1/1
  Sum2/1 -> Unbuffer/1
  x/1 -> Buffer/1
  Constant/1 -> Sum1/2
  Product/1 -> Sum2/2
  Buffer/1 -> Sum/1, Unit Delay/1
  Unbuffer/1 -> Out1/1

== system KPA_ALL/Symbol synchronization1/Loop filter ==
  In1 : Inport
  Out1 : Outport
  wires:
  In1/1 -> Out1/1

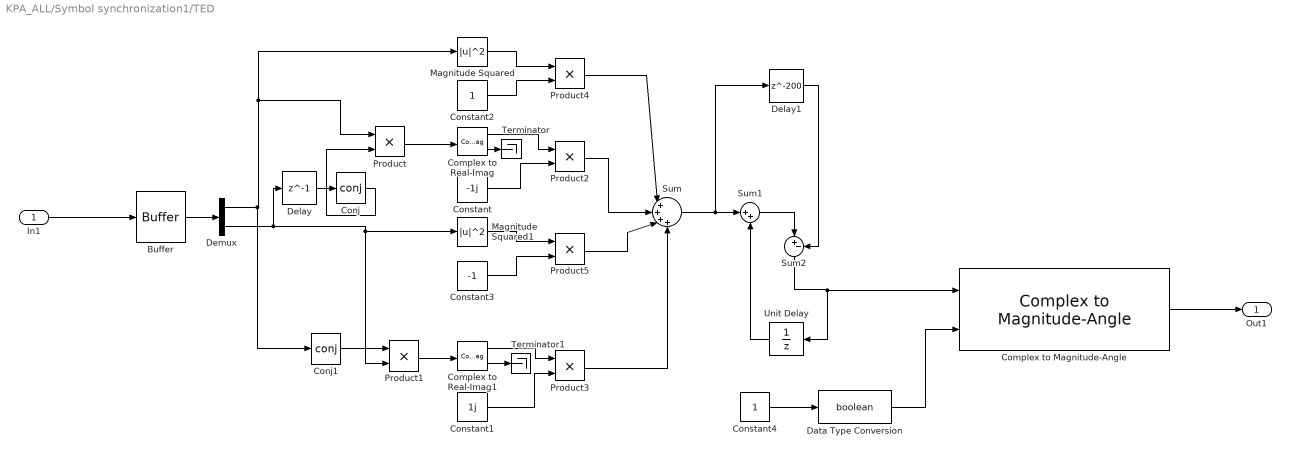
== system KPA_ALL/Symbol synchronization1/TED ==
  In1 : Inport
  Buffer : Buffer  N=2  OutputFrames=off
  Complex to Real-Imag : ComplexToRealImag
  Complex to Real-Imag1 : ComplexToRealImag
  Complex to Magnitude-Angle : dsphdlmathfun2/Complex to Magnitude-Angle  NumIterationsSource=Auto  NumIterations=10  OutputFormat=Magnitude and angle  AngleFormat=Normalized  ScaleOutput=on  ScalingMethod=Shift-Add  SimulateUsing=Code generation
  Conj : Math  Operator=conj
  Conj1 : Math  Operator=conj
  Constant : Constant  Value=-1j
  Constant1 : Constant  Value=1j
  Constant2 : Constant
  Constant3 : Constant  Value=-1
  Constant4 : Constant  SampleTime=-1
  Data Type Conversion : DataTypeConversion  OutDataTypeStr=boolean  SaturateOnIntegerOverflow=off  RndMeth=Floor
  Delay : Delay  DelayLength=1  InitialCondition=0
  Delay1 : Delay  DelayLength=200
  Demux : Demux  Outputs=2
  Magnitude Squared : Math  Operator=magnitude^2
  Magnitude Squared1 : Math  Operator=magnitude^2
  Product{,1..5} (6 alike) : Product
  Sum : Sum  Inputs=|++++
  Sum1 : Sum  Inputs=|++
  Sum2 : Sum  Inputs=|+-
  Terminator : Terminator
  Terminator1 : Terminator
  Unit Delay : UnitDelay  SampleTime=-1  HasFrameUpgradeWarning=on
  Out1 : Outport
  wires:
  In1/1 -> Buffer/1
  Complex to Magnitude-Angle/2 -> Out1/1
  Product4/1 -> Sum/1
  Complex to Real-Imag1/2 -> Terminator1/1
  Sum1/1 -> Sum2/1
  Constant1/1 -> Product3/2
  Product3/1 -> Sum/4
  Conj/1 -> Product/2
  Complex to Real-Imag/2 -> Terminator/1
  Conj1/1 -> Product1/1
  Delay1/1 -> Sum2/2
  Delay/1 -> Conj/1
  Sum2/1 -> Unit Delay/1, Complex to Magnitude-Angle/1
  Constant4/1 -> Data Type Conversion/1
  Constant3/1 -> Product5/2
  Sum/1 -> Sum1/1, Delay1/1
  Complex to Real-Imag1/1 -> Product3/1
  Product/1 -> Complex to Real-Imag/1
  Product1/1 -> Complex to Real-Imag1/1
  Complex to Real-Imag/1 -> Product2/1
  Magnitude Squared1/1 -> Product5/1
  Constant/1 -> Product2/2
  Unit Delay/1 -> Sum1/2
  Constant2/1 -> Product4/2
  Product2/1 -> Sum/2
  Buffer/1 -> Demux/1
  Product5/1 -> Sum/3
  Demux/2 -> Delay/1, Product1/2, Magnitude Squared1/1
  Magnitude Squared/1 -> Product4/1
  Demux/1 -> Conj1/1, Product/1, Magnitude Squared/1
  Data Type Conversion/1 -> Complex to Magnitude-Angle/2

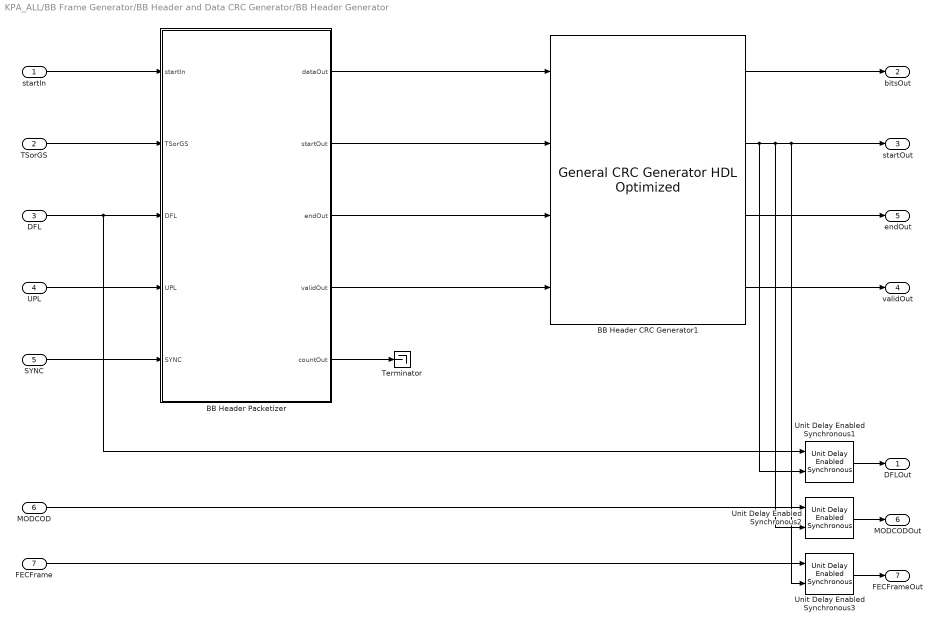
== system KPA_ALL/BB Frame Generator/BB Header and Data CRC Generator/BB Header Generator ==
  startIn : Inport
  TSorGS : Inport  Port=2
  DFL : Inport  Port=3
  UPL : Inport  Port=4
  SYNC : Inport  Port=5
  MODCOD : Inport  Port=6
  FECFrame : Inport  Port=7
  BB Header CRC Generator1 : commhdlcrc/General CRC Generator HDL Optimized  Polynomial=[1 1 1 0 1 0 1 0 1]  InitialState=0  DirectMethod=off  ReflectInput=off  ReflectCRCChecksum=off  FinalXORValue=0  SimulateUsing=Code generation
  BB Header Packetizer : MATLAB Function  TreatAsAtomicUnit=on
  Terminator : Terminator
  Unit Delay Enabled Synchronous1 : hdlsllib/Discrete/Unit Delay Enabled Synchronous  InitialCondition=0.0  SampleTime=-1
  Unit Delay Enabled Synchronous2 : hdlsllib/Discrete/Unit Delay Enabled Synchronous  InitialCondition=0.0  SampleTime=-1
  Unit Delay Enabled Synchronous3 : hdlsllib/Discrete/Unit Delay Enabled Synchronous  InitialCondition=0.0  SampleTime=-1
  DFLOut : Outport
  bitsOut : Outport  Port=2
  startOut : Outport  Port=3
  validOut : Outport  Port=4
  endOut : Outport  Port=5
  MODCODOut : Outport  Port=6
  FECFrameOut : Outport  Port=7
  wires:
  startIn/1 -> BB Header Packetizer/1(startIn)
  TSorGS/1 -> BB Header Packetizer/2(TSorGS)
  UPL/1 -> BB Header Packetizer/4(UPL)
  FECFrame/1 -> Unit Delay Enabled Synchronous3/1
  DFL/1 -> Unit Delay Enabled Synchronous1/1, BB Header Packetizer/3(DFL)
  SYNC/1 -> BB Header Packetizer/5(SYNC)
  BB Header CRC Generator1/2 -> Unit Delay Enabled Synchronous1/2, Unit Delay Enabled Synchronous2/2, Unit Delay Enabled Synchronous3/2, startOut/1
  BB Header CRC Generator1/4 -> validOut/1
  Unit Delay Enabled Synchronous2/1 -> MODCODOut/1
  BB Header CRC Generator1/1 -> bitsOut/1
  Unit Delay Enabled Synchronous1/1 -> DFLOut/1
  Unit Delay Enabled Synchronous3/1 -> FECFrameOut/1
  BB Header CRC Generator1/3 -> endOut/1
  BB Header Packetizer/4(validOut) -> BB Header CRC Generator1/4
  BB Header Packetizer/3(endOut) -> BB Header CRC Generator1/3
  BB Header Packetizer/2(startOut) -> BB Header CRC Generator1/2
  BB Header Packetizer/1(dataOut) -> BB Header CRC Generator1/1
  BB Header Packetizer/5(countOut) -> Terminator/1
  MODCOD/1 -> Unit Delay Enabled Synchronous2/1

== system KPA_ALL/BB Frame Generator/BB Header and Data CRC Generator/Data Field Generator ==
  note: UPL is a logical signal that describes whether the data should be treated as packets or as continuous stream. Currently only continuous stream is supported in the model.
  dataIn : Inport
  validIn : Inport  Port=2
  frameEnd : Inport  Port=3
  frameStart : Inport  Port=4
  UPL : Inport  Port=5
  Delay{,1..3} (4 alike) : Delay  DelayLength=1
  Terminator : Terminator
  dataOut : Outport
  validOut : Outport  Port=2
  frameEndOut : Outport  Port=3
  frameStartOut : Outport  Port=4
  wires:
  frameEnd/1 -> Delay2/1
  dataIn/1 -> Delay/1
  frameStart/1 -> Delay3/1
  Delay/1 -> dataOut/1
  Delay1/1 -> validOut/1
  Delay2/1 -> frameEndOut/1
  Delay3/1 -> frameStartOut/1
  validIn/1 -> Delay1/1
  UPL/1 -> Terminator/1

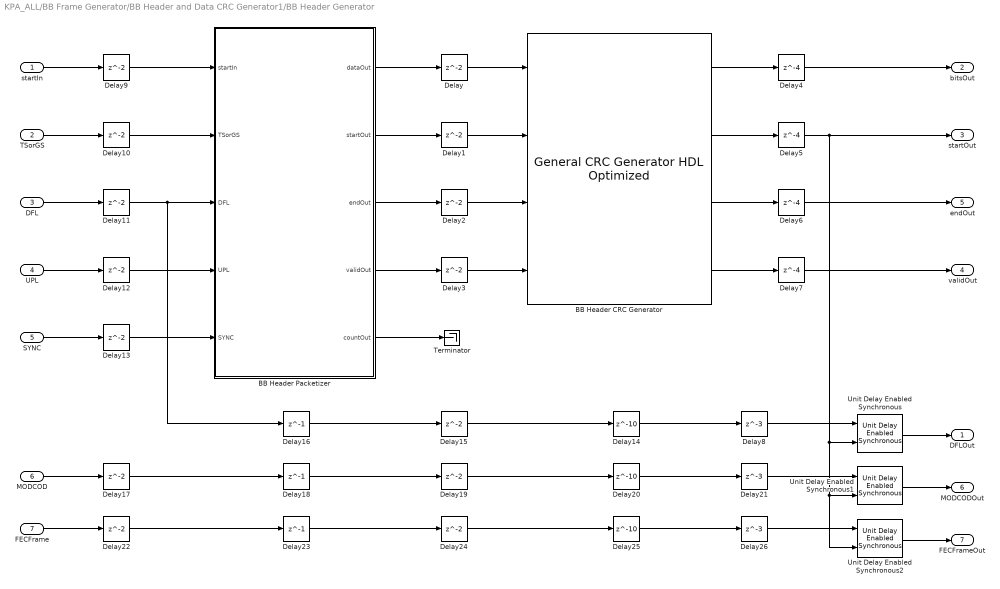
== system KPA_ALL/BB Frame Generator/BB Header and Data CRC Generator1/BB Header Generator ==
  startIn : Inport
  TSorGS : Inport  Port=2
  DFL : Inport  Port=3
  UPL : Inport  Port=4
  SYNC : Inport  Port=5
  MODCOD : Inport  Port=6
  FECFrame : Inport  Port=7
  BB Header CRC Generator : commhdlcrc/General CRC Generator HDL Optimized  Polynomial=[1 1 1 0 1 0 1 0 1]  InitialState=0  DirectMethod=off  ReflectInput=off  ReflectCRCChecksum=off  FinalXORValue=0  SimulateUsing=Code generation
  BB Header Packetizer : MATLAB Function  TreatAsAtomicUnit=on
  Delay{,1..3,9..13,15,17,19,22,24} (14 alike) : Delay
  Delay14 : Delay  DelayLength=10
  Delay16 : Delay  DelayLength=1
  Delay18 : Delay  DelayLength=1
  Delay20 : Delay  DelayLength=10
  Delay21 : Delay  DelayLength=3
  Delay23 : Delay  DelayLength=1
  Delay25 : Delay  DelayLength=10
  Delay26 : Delay  DelayLength=3
  Delay{4..7} (4 alike) : Delay  DelayLength=4
  Delay8 : Delay  DelayLength=3
  Terminator : Terminator
  Unit Delay Enabled Synchronous : hdlsllib/Discrete/Unit Delay Enabled Synchronous  InitialCondition=0.0  SampleTime=-1
  Unit Delay Enabled Synchronous1 : hdlsllib/Discrete/Unit Delay Enabled Synchronous  InitialCondition=0.0  SampleTime=-1
  Unit Delay Enabled Synchronous2 : hdlsllib/Discrete/Unit Delay Enabled Synchronous  InitialCondition=0.0  SampleTime=-1
  DFLOut : Outport
  bitsOut : Outport  Port=2
  startOut : Outport  Port=3
  validOut : Outport  Port=4
  endOut : Outport  Port=5
  MODCODOut : Outport  Port=6
  FECFrameOut : Outport  Port=7
  wires:
  TSorGS/1 -> Delay10/1
  SYNC/1 -> Delay13/1
  BB Header Packetizer/3(endOut) -> Delay2/1
  BB Header Packetizer/2(startOut) -> Delay1/1
  BB Header Packetizer/4(validOut) -> Delay3/1
  DFL/1 -> Delay11/1
  startIn/1 -> Delay9/1
  BB Header Packetizer/1(dataOut) -> Delay/1
  BB Header CRC Generator/1 -> Delay4/1
  UPL/1 -> Delay12/1
  BB Header CRC Generator/2 -> Delay5/1
  BB Header CRC Generator/4 -> Delay7/1
  BB Header CRC Generator/3 -> Delay6/1
  BB Header Packetizer/5(countOut) -> Terminator/1
  Delay/1 -> BB Header CRC Generator/1
  Delay1/1 -> BB Header CRC Generator/2
  Delay2/1 -> BB Header CRC Generator/3
  Delay3/1 -> BB Header CRC Generator/4
  Delay4/1 -> bitsOut/1
  Delay6/1 -> endOut/1
  Delay7/1 -> validOut/1
  Delay9/1 -> BB Header Packetizer/1(startIn)
  Delay10/1 -> BB Header Packetizer/2(TSorGS)
  Delay12/1 -> BB Header Packetizer/4(UPL)
  Delay13/1 -> BB Header Packetizer/5(SYNC)
  Delay8/1 -> Unit Delay Enabled Synchronous/1
  Delay14/1 -> Delay8/1
  Delay15/1 -> Delay14/1
  Delay11/1 -> BB Header Packetizer/3(DFL), Delay16/1
  Delay16/1 -> Delay15/1
  Unit Delay Enabled Synchronous/1 -> DFLOut/1
  Delay5/1 -> startOut/1, Unit Delay Enabled Synchronous2/2, Unit Delay Enabled Synchronous1/2, Unit Delay Enabled Synchronous/2
  MODCOD/1 -> Delay17/1
  Delay17/1 -> Delay18/1
  Delay18/1 -> Delay19/1
  Delay19/1 -> Delay20/1
  Delay20/1 -> Delay21/1
  Delay21/1 -> Unit Delay Enabled Synchronous1/1
  Unit Delay Enabled Synchronous1/1 -> MODCODOut/1
  FECFrame/1 -> Delay22/1
  Unit Delay Enabled Synchronous2/1 -> FECFrameOut/1
  Delay22/1 -> Delay23/1
  Delay23/1 -> Delay24/1
  Delay24/1 -> Delay25/1
  Delay25/1 -> Delay26/1
  Delay26/1 -> Unit Delay Enabled Synchronous2/1

== system KPA_ALL/BB Frame Generator/BB Header and Data CRC Generator1/Data Field Generator ==
  dataIn : Inport
  startIn : Inport  Port=2
  endIn : Inport  Port=3
  validIn : Inport  Port=4
  frameEnd : Inport  Port=5
  frameStart : Inport  Port=6
  UPL : Inport  Port=7
  Compare To Constant : simulink/Logic and Bit Operations/Compare To Constant  relop=~=  const=0  OutDataTypeStr=boolean
  Continuous Streams : Subsystem
  Packetized Streams : Subsystem
  Switch{,1..3} (4 alike) : Switch  Criteria=u2 ~= 0  SaturateOnIntegerOverflow=off  InputSameDT=off
  pktBits : Outport
  pktValid : Outport  Port=2
  frameStartOut : Outport  Port=3
  frameEndOut : Outport  Port=4
  wires:
  dataIn/1 -> Continuous Streams/1(dataIn), Packetized Streams/1(dataIn)
  startIn/1 -> Packetized Streams/2(startIn)
  endIn/1 -> Packetized Streams/3(endIn)
  validIn/1 -> Continuous Streams/2(validIn), Packetized Streams/4(validIn)
  Packetized Streams/1(pktBits) -> Switch/1
  Packetized Streams/2(pktValid) -> Switch1/1
  Packetized Streams/3(frameEndOut) -> Switch2/1
  Packetized Streams/4(frameStartOut) -> Switch3/1
  Switch/1 -> pktBits/1
  Switch1/1 -> pktValid/1
  Switch2/1 -> frameEndOut/1
  Switch3/1 -> frameStartOut/1
  Continuous Streams/3(frameEndOut) -> Switch2/3
  Continuous Streams/4(frameStartOut) -> Switch3/3
  Continuous Streams/2(validOut) -> Switch1/3
  Continuous Streams/1(dataOut) -> Switch/3
  frameEnd/1 -> Continuous Streams/3(frameEnd), Packetized Streams/5(frameEnd)
  frameStart/1 -> Continuous Streams/4(frameStart), Packetized Streams/6(frameStart)
  UPL/1 -> Compare To Constant/1
  Compare To Constant/1 -> Switch3/2, Switch2/2, Switch1/2, Switch/2

== system KPA_ALL/BB Frame Generator/BB Scrambler/Subsystem ==
  In1 : Inport
  Enable : EnablePort
  PN Sequence Generator : commseqgen3/PN Sequence Generator  poly='z^15 + z + 1'  ini_sta=[1 0 0 1 0 1 0 1 0 0 0 0 0 0 0]  outBitMaskSource=Dialog parameter  shift=15  outVarSiz=off  maxOutSizeMode=Dialog parameter  maxOutSize=[10 1]  Ts=-1  sampPerFrame=1  reset=on  bitPackedOutputs=off  outDataType=Smallest unsigned integer  numPackedBits=8  bitPackDataSigned=off  bitPackedOutDType=double
  Out1 : Outport  InitialOutput=0
  wires:
  In1/1 -> PN Sequence Generator/1
  PN Sequence Generator/1 -> Out1/1

== system KPA_ALL/BB Frame Generator/Data Store FIFO/No HDL ==
  wr : Inport
  full : Inport  Port=2
  ncount : Inport  Port=3
  empty : Inport  Port=4
  rd : Inport  Port=5
  Assertion : Assertion  AssertionFailFcn=warning('push on to a full RAM');  StopWhenAssertionFail=off
  Assertion1 : Assertion  AssertionFailFcn=warning('pop from an empty RAM');  StopWhenAssertionFail=off
  Display : Display
  Logical Operator : Logic  Operator=NAND  AllPortsSameDT=off  OutDataTypeStr=boolean
  Logical Operator1 : Logic  Operator=NAND  AllPortsSameDT=off  OutDataTypeStr=boolean
  wires:
  rd/1 -> Logical Operator1/2
  Logical Operator/1 -> Assertion/1
  empty/1 -> Logical Operator1/1
  ncount/1 -> Display/1
  full/1 -> Logical Operator/2
  wr/1 -> Logical Operator/1
  Logical Operator1/1 -> Assertion1/1

== system KPA_ALL/BB Frame Generator/Multiplexer/No HDL ==
  In1 : Inport
  In2 : Inport  Port=2
  Assertion : Assertion
  Logical Operator1 : Logic  AllPortsSameDT=off  OutDataTypeStr=boolean
  Logical Operator2 : Logic  Operator=NOT  AllPortsSameDT=off  OutDataTypeStr=boolean
  wires:
  Logical Operator2/1 -> Assertion/1
  In2/1 -> Logical Operator1/2
  Logical Operator1/1 -> Logical Operator2/1
  In1/1 -> Logical Operator1/1

== system KPA_ALL/BB Frame Generator/BB Header and Data CRC Generator1/Data Field Generator/Continuous Streams ==
  dataIn : Inport
  validIn : Inport  Port=2
  frameEnd : Inport  Port=3
  frameStart : Inport  Port=4
  Delay{,1..3} (4 alike) : Delay  DelayLength=8+1+10
  dataOut : Outport
  validOut : Outport  Port=2
  frameEndOut : Outport  Port=3
  frameStartOut : Outport  Port=4
  wires:
  Delay/1 -> dataOut/1
  dataIn/1 -> Delay/1
  Delay1/1 -> validOut/1
  frameStart/1 -> Delay3/1
  Delay3/1 -> frameStartOut/1
  Delay2/1 -> frameEndOut/1
  frameEnd/1 -> Delay2/1
  validIn/1 -> Delay1/1
